simulink model "CrCtl_Governor"  (R2016b)
settings: configuration reference "CodeGenConfigSet" (kept outside this file)
values from neighbouring files (symbols this model uses):
  ACC_ZERO = fi(0,Acc_m_s2)    [init_CrCtl_Governor.m]
  CrCtl_facAcc2TrqCor_C = Calibration.Parameter    [init_CrCtl_Governor.m]
  CrCtl_facDecl2TrqCor_C = Calibration.Parameter    [init_CrCtl_Governor.m]
  CrCtl_facPT11_C = Calibration.Parameter    [init_CrCtl_Governor.m]
  CrCtl_facPT12_C = Calibration.Parameter    [init_CrCtl_Governor.m]
  CrCtl_facPT13_C = Calibration.Parameter    [init_CrCtl_Governor.m]
  CrCtl_facRmpSlpHiAcc_C = Calibration.Parameter    [init_CrCtl_Governor.m]
  CrCtl_facRmpSlpHiDecl_C = Calibration.Parameter    [init_CrCtl_Governor.m]
  CrCtl_facSlpConstRmpDwn_C = Calibration.Parameter    [init_CrCtl_Governor.m]
  CrCtl_facSlpConstRmpUp_C = Calibration.Parameter    [init_CrCtl_Governor.m]
  CrCtl_facSlpRmp1Sus_C = Calibration.Parameter    [init_CrCtl_Governor.m]
  CrCtl_facSlpRmp2Sus_C = Calibration.Parameter    [init_CrCtl_Governor.m]
  CrCtl_facTipDwnCor_CUR = Calibration.Parameter    [init_CrCtl_Governor.m]
  CrCtl_facTipDwnCor_CURX = Calibration.Parameter    [init_CrCtl_Governor.m]
  CrCtl_facTipUpCor_CUR = Calibration.Parameter    [init_CrCtl_Governor.m]
  CrCtl_facTipUpCor_CURX = Calibration.Parameter    [init_CrCtl_Governor.m]
  CrCtl_facTrqIncrSlpConstRmp_C = Calibration.Parameter    [init_CrCtl_Governor.m]
  CrCtl_facTrqIncrTimeConstRmp_C = Calibration.Parameter    [init_CrCtl_Governor.m]
  CrCtl_facTrqRedSlpConstRmp_C = Calibration.Parameter    [init_CrCtl_Governor.m]
  CrCtl_facTrqRedTimeConstRmp_C = Calibration.Parameter    [init_CrCtl_Governor.m]
  CrCtl_facTrqStrtAcc_C = Calibration.Parameter    [init_CrCtl_Governor.m]
  CrCtl_KiAcc1IWin_C = Calibration.Parameter    [init_CrCtl_Governor.m]
  CrCtl_KiAcc2IWin_C = Calibration.Parameter    [init_CrCtl_Governor.m]
  CrCtl_KiAcc3IWin_C = Calibration.Parameter    [init_CrCtl_Governor.m]
  CrCtl_KiCruise1IWin_C = Calibration.Parameter    [init_CrCtl_Governor.m]
  CrCtl_KiCruise2IWin_C = Calibration.Parameter    [init_CrCtl_Governor.m]
  CrCtl_KiCruise3IWin_C = Calibration.Parameter    [init_CrCtl_Governor.m]
  CrCtl_KiDecl1IWin_C = Calibration.Parameter    [init_CrCtl_Governor.m]
  CrCtl_KiDecl2IWin_C = Calibration.Parameter    [init_CrCtl_Governor.m]
  CrCtl_KiDecl3IWin_C = Calibration.Parameter    [init_CrCtl_Governor.m]
  CrCtl_KiNegAcc1IWin_C = Calibration.Parameter    [init_CrCtl_Governor.m]
  CrCtl_KiNegAcc2IWin_C = Calibration.Parameter    [init_CrCtl_Governor.m]
  CrCtl_KiNegAcc3IWin_C = Calibration.Parameter    [init_CrCtl_Governor.m]
  CrCtl_KiNegCruise1IWin_C = Calibration.Parameter    [init_CrCtl_Governor.m]
  CrCtl_KiNegCruise2IWin_C = Calibration.Parameter    [init_CrCtl_Governor.m]
  CrCtl_KiNegCruise3IWin_C = Calibration.Parameter    [init_CrCtl_Governor.m]
  CrCtl_KiNegDecl1IWin_C = Calibration.Parameter    [init_CrCtl_Governor.m]
  CrCtl_KiNegDecl2IWin_C = Calibration.Parameter    [init_CrCtl_Governor.m]
  CrCtl_KiNegDecl3IWin_C = Calibration.Parameter    [init_CrCtl_Governor.m]
  CrCtl_KiNegRes1IWin_C = Calibration.Parameter    [init_CrCtl_Governor.m]
  CrCtl_KiNegRes2IWin_C = Calibration.Parameter    [init_CrCtl_Governor.m]
  CrCtl_KiNegRes3IWin_C = Calibration.Parameter    [init_CrCtl_Governor.m]
  CrCtl_KiNegResCruise1IWin_C = Calibration.Parameter    [init_CrCtl_Governor.m]
  CrCtl_KiNegResCruise2IWin_C = Calibration.Parameter    [init_CrCtl_Governor.m]
  CrCtl_KiNegResCruise3IWin_C = Calibration.Parameter    [init_CrCtl_Governor.m]
  CrCtl_KiPosAcc1IWin_C = Calibration.Parameter    [init_CrCtl_Governor.m]
  CrCtl_KiPosAcc2IWin_C = Calibration.Parameter    [init_CrCtl_Governor.m]
  CrCtl_KiPosAcc3IWin_C = Calibration.Parameter    [init_CrCtl_Governor.m]
  CrCtl_KiPosCruise1IWin_C = Calibration.Parameter    [init_CrCtl_Governor.m]
  CrCtl_KiPosCruise2IWin_C = Calibration.Parameter    [init_CrCtl_Governor.m]
  CrCtl_KiPosCruise3IWin_C = Calibration.Parameter    [init_CrCtl_Governor.m]
  CrCtl_KiPosDecl1IWin_C = Calibration.Parameter    [init_CrCtl_Governor.m]
  CrCtl_KiPosDecl2IWin_C = Calibration.Parameter    [init_CrCtl_Governor.m]
  CrCtl_KiPosDecl3IWin_C = Calibration.Parameter    [init_CrCtl_Governor.m]
  CrCtl_KiPosRes1IWin_C = Calibration.Parameter    [init_CrCtl_Governor.m]
  CrCtl_KiPosRes3IWin_C = Calibration.Parameter    [init_CrCtl_Governor.m]
  CrCtl_KiPosResCruise1IWin_C = Calibration.Parameter    [init_CrCtl_Governor.m]
  CrCtl_KiPosResCruise2IWin_C = Calibration.Parameter    [init_CrCtl_Governor.m]
  CrCtl_KiPosResCruise3IWin_C = Calibration.Parameter    [init_CrCtl_Governor.m]
  CrCtl_KiRes1IWin_C = Calibration.Parameter    [init_CrCtl_Governor.m]
  CrCtl_KiRes2IWin_C = Calibration.Parameter    [init_CrCtl_Governor.m]
  CrCtl_KiRes3IWin_C = Calibration.Parameter    [init_CrCtl_Governor.m]
  CrCtl_KiResCruise1IWin_C = Calibration.Parameter    [init_CrCtl_Governor.m]
  CrCtl_KiResCruise2IWin_C = Calibration.Parameter    [init_CrCtl_Governor.m]
  CrCtl_KiResCruise3IWin_C = Calibration.Parameter    [init_CrCtl_Governor.m]
  CrCtl_KpAcc1PWin_C = Calibration.Parameter    [init_CrCtl_Governor.m]
  CrCtl_KpAcc2PWin_C = Calibration.Parameter    [init_CrCtl_Governor.m]
  CrCtl_KpAcc3PWin_C = Calibration.Parameter    [init_CrCtl_Governor.m]
  CrCtl_KpCruise1PWin_C = Calibration.Parameter    [init_CrCtl_Governor.m]
  CrCtl_KpCruise2PWin_C = Calibration.Parameter    [init_CrCtl_Governor.m]
  CrCtl_KpCruise3PWin_C = Calibration.Parameter    [init_CrCtl_Governor.m]
  CrCtl_KpDecl1PWin_C = Calibration.Parameter    [init_CrCtl_Governor.m]
  CrCtl_KpDecl2PWin_C = Calibration.Parameter    [init_CrCtl_Governor.m]
  CrCtl_KpDecl3PWin_C = Calibration.Parameter    [init_CrCtl_Governor.m]
  CrCtl_KpNegAcc1PWin_C = Calibration.Parameter    [init_CrCtl_Governor.m]
  CrCtl_KpNegAcc2PWin_C = Calibration.Parameter    [init_CrCtl_Governor.m]
  CrCtl_KpNegAcc3PWin_C = Calibration.Parameter    [init_CrCtl_Governor.m]
  CrCtl_KpNegCruise1PWin_C = Calibration.Parameter    [init_CrCtl_Governor.m]
  CrCtl_KpNegCruise2PWin_C = Calibration.Parameter    [init_CrCtl_Governor.m]
  CrCtl_KpNegCruise3PWin_C = Calibration.Parameter    [init_CrCtl_Governor.m]
  CrCtl_KpNegDecl1PWin_C = Calibration.Parameter    [init_CrCtl_Governor.m]
  CrCtl_KpNegDecl2PWin_C = Calibration.Parameter    [init_CrCtl_Governor.m]
  CrCtl_KpNegDecl3PWin_C = Calibration.Parameter    [init_CrCtl_Governor.m]
  CrCtl_KpNegRes1PWin_C = Calibration.Parameter    [init_CrCtl_Governor.m]
  CrCtl_KpNegRes2PWin_C = Calibration.Parameter    [init_CrCtl_Governor.m]
  CrCtl_KpNegRes3PWin_C = Calibration.Parameter    [init_CrCtl_Governor.m]
  CrCtl_KpNegResCruise1PWin_C = Calibration.Parameter    [init_CrCtl_Governor.m]
  CrCtl_KpNegResCruise2PWin_C = Calibration.Parameter    [init_CrCtl_Governor.m]
  CrCtl_KpNegResCruise3PWin_C = Calibration.Parameter    [init_CrCtl_Governor.m]
  CrCtl_KpPosAcc1PWin_C = Calibration.Parameter    [init_CrCtl_Governor.m]
  CrCtl_KpPosAcc2PWin_C = Calibration.Parameter    [init_CrCtl_Governor.m]
  CrCtl_KpPosAcc3PWin_C = Calibration.Parameter    [init_CrCtl_Governor.m]
  CrCtl_KpPosCruise1PWin_C = Calibration.Parameter    [init_CrCtl_Governor.m]
  CrCtl_KpPosCruise2PWin_C = Calibration.Parameter    [init_CrCtl_Governor.m]
  CrCtl_KpPosCruise3PWin_C = Calibration.Parameter    [init_CrCtl_Governor.m]
  CrCtl_KpPosDecl1PWin_C = Calibration.Parameter    [init_CrCtl_Governor.m]
  CrCtl_KpPosDecl2PWin_C = Calibration.Parameter    [init_CrCtl_Governor.m]
  CrCtl_KpPosDecl3PWin_C = Calibration.Parameter    [init_CrCtl_Governor.m]
  CrCtl_KpPosRes1PWin_C = Calibration.Parameter    [init_CrCtl_Governor.m]
  CrCtl_KpPosRes2PWin_C = Calibration.Parameter    [init_CrCtl_Governor.m]
  CrCtl_KpPosRes3PWin_C = Calibration.Parameter    [init_CrCtl_Governor.m]
  CrCtl_KpPosResCruise1PWin_C = Calibration.Parameter    [init_CrCtl_Governor.m]
  CrCtl_KpPosResCruise2PWin_C = Calibration.Parameter    [init_CrCtl_Governor.m]
  CrCtl_KpPosResCruise3PWin_C = Calibration.Parameter    [init_CrCtl_Governor.m]
  CrCtl_KpRes1PWin_C = Calibration.Parameter    [init_CrCtl_Governor.m]
  CrCtl_KpRes2PWin_C = Calibration.Parameter    [init_CrCtl_Governor.m]
  CrCtl_KpRes3PWin_C = Calibration.Parameter    [init_CrCtl_Governor.m]
  CrCtl_KpResCruise1PWin_C = Calibration.Parameter    [init_CrCtl_Governor.m]
  CrCtl_KpResCruise2PWin_C = Calibration.Parameter    [init_CrCtl_Governor.m]
  CrCtl_KpResCruise3PWin_C = Calibration.Parameter    [init_CrCtl_Governor.m]
  CrCtl_numParSelThres1_C = Calibration.Parameter    [init_CrCtl_Governor.m]
  CrCtl_numParSelThres2_C = Calibration.Parameter    [init_CrCtl_Governor.m]
  CrCtl_swtBrkMode_C = Calibration.Parameter    [init_CrCtl_Governor.m]
  CrCtl_swtILimWithP_C = Calibration.Parameter    [init_CrCtl_Governor.m]
  CrCtl_swtOvrRdeFrzInteg_C = Calibration.Parameter    [init_CrCtl_Governor.m]
  CrCtl_swtParSelHysBrk_C = Calibration.Parameter    [init_CrCtl_Governor.m]
  CrCtl_swtPT1EngBrk_C = Calibration.Parameter    [init_CrCtl_Governor.m]
  CrCtl_swtSusRmpInit_C = Calibration.Parameter    [init_CrCtl_Governor.m]
  CrCtl_swtSusRmpStp_C = Calibration.Parameter    [init_CrCtl_Governor.m]
  CrCtl_swtTipUpDwnGvnrStrtVal_C = Calibration.Parameter    [init_CrCtl_Governor.m]
  ... (+88 more)
undefined symbols (not defined in the file or in its folder): CrCtl_Governor_DT, CrCtl_stLck_conv, CrCtl_stOpFunc_conv, CrCtl_stShOff_conv, CrCtl_stSub_conv, CrCtl_stSuspRamp_conv, CruiseCtl_State_conv, EBrk_stPreSelMode_conv, WESDem_State_conv
libraries: CXLib x126, simulink x25
(part 2 of 6)

== system CrCtl_Governor/OFF State ==
  CrCtl_trqLimAct : Inport
  CrCtl_trqMin : Inport  Port=2
  CrCtl_stShOff : Inport  Port=3
  PT_trqWhlMinEng : Inport  Port=4
  CrCtl_trqReqOld : Inport  Port=5
  CrCtl_stSubGvnr : Inport  Port=6
  CrCtl_st : Inport  Port=7
  CrCtl_stSub : Inport  Port=8
  CrCtl_stLck : Inport  Port=9
  Enable : EnablePort
  CRCTL_SUBRMP : Subsystem
  "CRCTL_SUBSTRTVAL " : Subsystem
  Constant1 : Constant  Value=CrCtl_stSub_conv.CRCTL_SUBRMP
  Constant2 : Constant  Value=CrCtl_stSub_conv.CRCTL_SUBSTRTVAL
  Merge : Merge
  Relational Operator1 : RelationalOperator  Operator===  OutDataTypeStr=boolean  RndMeth=Simplest
  Relational Operator2 : RelationalOperator  Operator===  OutDataTypeStr=boolean  RndMeth=Simplest
  Terminator : Terminator
  Terminator1 : Terminator
  Terminator2 : Terminator
  CrCtl_trqReq : Outport
  wires:
  CrCtl_trqLimAct/1 -> CRCTL_SUBRMP/4(CrCtl_trqLimAct), "CRCTL_SUBSTRTVAL "/1(CrCtl_trqLimAct)
  CrCtl_trqMin/1 -> CRCTL_SUBRMP/5(CrCtl_trqMin), "CRCTL_SUBSTRTVAL "/2(CrCtl_trqMin)
  Constant2/1 -> Relational Operator2/2
  Relational Operator2/1 -> "CRCTL_SUBSTRTVAL "/Enable
  CrCtl_stSubGvnr/1 -> Relational Operator1/1, Relational Operator2/1
  Constant1/1 -> Relational Operator1/2
  Relational Operator1/1 -> CRCTL_SUBRMP/Enable
  CrCtl_st/1 -> CRCTL_SUBRMP/1(CrCtl_st)
  CrCtl_stSub/1 -> CRCTL_SUBRMP/2(CrCtl_stSub)
  CrCtl_stLck/1 -> CRCTL_SUBRMP/3(CrCtl_stLck)
  Merge/1 -> CrCtl_trqReq/1
  "CRCTL_SUBSTRTVAL "/1(CrCtl_trqReq) -> Merge/1
  CRCTL_SUBRMP/4(CrCtl_trqReq) -> Merge/2
  CRCTL_SUBRMP/1(CrCtl_st_mp) -> Terminator/1
  CRCTL_SUBRMP/3(CrCtl_stLck_mp) -> Terminator2/1
  CRCTL_SUBRMP/2(CrCtl_stSub_mp) -> Terminator1/1
  PT_trqWhlMinEng/1 -> CRCTL_SUBRMP/7(PT_trqWhlMinEng)
  CrCtl_stShOff/1 -> CRCTL_SUBRMP/6(CrCtl_stShOff)
  CrCtl_trqReqOld/1 -> "CRCTL_SUBSTRTVAL "/3(CrCtl_trqReqOld), CRCTL_SUBRMP/8(CrCtl_trqReqOld)

== system CrCtl_Governor/Operating Status Cruise Control ==
  CrCtl_stGvnr : Inport
  CrCtl_stSubGvnr : Inport  Port=2
  CrCtl_stShOff : Inport  Port=3
  CrCtl_stIWin_mp : Inport  Port=4
  Bitwise Operator : simulink/Logic and Bit Operations/Bitwise Operator  logicop=AND  UseBitMask=on  BitMask=bin2dec('00000010')  BitMaskRealWorld=Stored Integer
  Constant : Constant  Value=CrCtl_stShOff_conv.CRCTL_CUT
  Constant1 : Constant  Value=CruiseCtl_State_conv.CrCtl_STAND_BY
  Constant2 : Constant  Value=CruiseCtl_State_conv.CrCtl_ERROR
  Constant3 : Constant  Value=CrCtl_stSub_conv.CRCTL_SUBNOSUB
  Constant4 : Constant  Value=CrCtl_stOpFunc_conv.CRCTL_NOTACTV
  Constant5 : Constant  Value=CrCtl_stOpFunc_conv.CRCTL_ACTV
  Constant6 : Constant  Value=CrCtl_stOpFunc_conv.CRCTL_OVERRIDE
  Constant7 : Constant  Value=CruiseCtl_State_conv.CrCtl_STAND_BY
  Constant9 : Constant  Value=CrCtl_stSub_conv.CRCTL_SUBNOSUB
  Logical Operator : Logic  AllPortsSameDT=off  OutDataTypeStr=boolean
  Logical Operator1 : Logic  Inputs=3  AllPortsSameDT=off  OutDataTypeStr=boolean
  Logical Operator2 : Logic  AllPortsSameDT=off  OutDataTypeStr=boolean
  Logical Operator3 : Logic  Inputs=3  AllPortsSameDT=off  OutDataTypeStr=boolean
  Relational Operator{,1..3} (4 alike) : RelationalOperator  Operator=~=  OutDataTypeStr=boolean  RndMeth=Simplest
  Relational Operator4 : RelationalOperator  Operator===  OutDataTypeStr=boolean  RndMeth=Simplest
  Relational Operator5 : RelationalOperator  Operator===  OutDataTypeStr=boolean  RndMeth=Simplest
  Switch : Switch  Criteria=u2 ~= 0
  Switch1 : Switch  Criteria=u2 ~= 0
  CrCtl_stReq : Outport
  CrCtl_stPtd : Outport  Port=2
  CrCtl_stOpFunc : Outport  Port=3
  wires:
  Constant1/1 -> Relational Operator/2
  Constant2/1 -> Relational Operator1/2
  CrCtl_stSubGvnr/1 -> Relational Operator5/1, Relational Operator2/1
  Constant3/1 -> Relational Operator2/2
  CrCtl_stShOff/1 -> Relational Operator3/1
  Constant/1 -> Relational Operator3/2
  Relational Operator/1 -> Logical Operator/1
  Relational Operator1/1 -> Logical Operator3/1, Logical Operator/2
  Logical Operator/1 -> Logical Operator1/1
  Relational Operator3/1 -> Logical Operator3/3, Logical Operator1/3
  Logical Operator1/1 -> CrCtl_stReq/1
  CrCtl_stIWin_mp/1 -> Bitwise Operator/1
  Bitwise Operator/1 -> Switch/2
  Constant6/1 -> Switch/1
  Switch1/1 -> Switch/3
  Switch/1 -> CrCtl_stOpFunc/1
  CrCtl_stGvnr/1 -> Relational Operator4/1, Relational Operator1/1, Relational Operator/1
  Constant7/1 -> Relational Operator4/2
  Relational Operator4/1 -> Logical Operator2/1
  Relational Operator5/1 -> Logical Operator2/2
  Constant9/1 -> Relational Operator5/2
  Logical Operator2/1 -> Switch1/2
  Constant4/1 -> Switch1/1
  Constant5/1 -> Switch1/3
  Relational Operator2/1 -> Logical Operator3/2, Logical Operator1/2
  Logical Operator3/1 -> CrCtl_stPtd/1

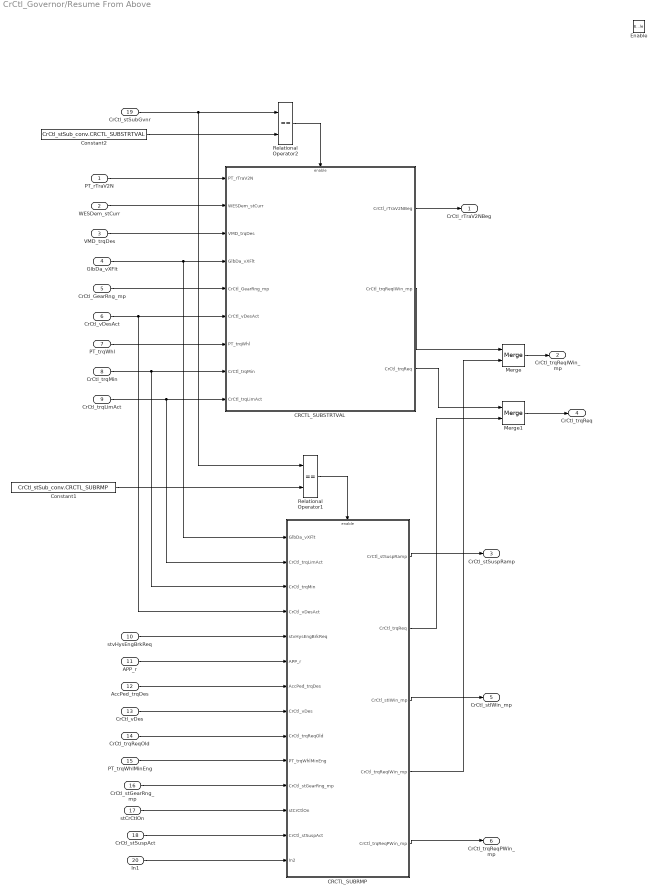
== system CrCtl_Governor/Resume From Above ==
  PT_rTraV2N : Inport
  WESDem_stCurr : Inport  Port=2
  VMD_trqDes : Inport  Port=3
  GlbDa_vXFlt : Inport  Port=4
  CrCtl_GearRng_mp : Inport  Port=5
  CrCtl_vDesAct : Inport  Port=6
  PT_trqWhl : Inport  Port=7
  CrCtl_trqMin : Inport  Port=8
  CrCtl_trqLimAct : Inport  Port=9
  stvHysEngBrkReq : Inport  Port=10
  APP_r : Inport  Port=11
  AccPed_trqDes : Inport  Port=12
  CrCtl_vDes : Inport  Port=13
  CrCtl_trqReqOld : Inport  Port=14
  PT_trqWhlMinEng : Inport  Port=15
  CrCtl_stGearRng_mp : Inport  Port=16
  stCrCtlOn : Inport  Port=17
  CrCtl_stSuspAct : Inport  Port=18
  CrCtl_stSubGvnr : Inport  Port=19
  In1 : Inport  Port=20
  Enable : EnablePort
  CRCTL_SUBRMP : Subsystem
  CRCTL_SUBSTRTVAL : Subsystem
  Constant1 : Constant  Value=CrCtl_stSub_conv.CRCTL_SUBRMP
  Constant2 : Constant  Value=CrCtl_stSub_conv.CRCTL_SUBSTRTVAL
  Merge : Merge
  Merge1 : Merge
  Relational Operator1 : RelationalOperator  Operator===  OutDataTypeStr=boolean  RndMeth=Simplest
  Relational Operator2 : RelationalOperator  Operator===  OutDataTypeStr=boolean  RndMeth=Simplest
  CrCtl_rTraV2NBeg : Outport
  CrCtl_trqReqIWin_mp : Outport  Port=2
  CrCtl_stSuspRamp : Outport  Port=3
  CrCtl_trqReq : Outport  Port=4
  CrCtl_stIWin_mp : Outport  Port=5
  CrCtl_trqReqPWin_mp : Outport  Port=6
  wires:
  PT_rTraV2N/1 -> CRCTL_SUBSTRTVAL/1(PT_rTraV2N)
  WESDem_stCurr/1 -> CRCTL_SUBSTRTVAL/2(WESDem_stCurr)
  VMD_trqDes/1 -> CRCTL_SUBSTRTVAL/3(VMD_trqDes)
  GlbDa_vXFlt/1 -> CRCTL_SUBRMP/1(GlbDa_vXFlt), CRCTL_SUBSTRTVAL/4(GlbDa_vXFlt)
  CrCtl_GearRng_mp/1 -> CRCTL_SUBSTRTVAL/5(CrCtl_GearRng_mp)
  CrCtl_trqLimAct/1 -> CRCTL_SUBRMP/2(CrCtl_trqLimAct), CRCTL_SUBSTRTVAL/9(CrCtl_trqLimAct)
  CrCtl_trqMin/1 -> CRCTL_SUBRMP/3(CrCtl_trqMin), CRCTL_SUBSTRTVAL/8(CrCtl_trqMin)
  PT_trqWhl/1 -> CRCTL_SUBSTRTVAL/7(PT_trqWhl)
  Constant2/1 -> Relational Operator2/2
  Relational Operator2/1 -> CRCTL_SUBSTRTVAL/Enable
  CrCtl_stSubGvnr/1 -> Relational Operator1/1, Relational Operator2/1
  Constant1/1 -> Relational Operator1/2
  Relational Operator1/1 -> CRCTL_SUBRMP/Enable
  CrCtl_vDesAct/1 -> CRCTL_SUBRMP/4(CrCtl_vDesAct), CRCTL_SUBSTRTVAL/6(CrCtl_vDesAct)
  stvHysEngBrkReq/1 -> CRCTL_SUBRMP/5(stvHysEngBrkReq)
  APP_r/1 -> CRCTL_SUBRMP/6(APP_r)
  AccPed_trqDes/1 -> CRCTL_SUBRMP/7(AccPed_trqDes)
  stCrCtlOn/1 -> CRCTL_SUBRMP/12(stCrCtlOn)
  CrCtl_stGearRng_mp/1 -> CRCTL_SUBRMP/11(CrCtl_stGearRng_mp)
  PT_trqWhlMinEng/1 -> CRCTL_SUBRMP/10(PT_trqWhlMinEng)
  CrCtl_vDes/1 -> CRCTL_SUBRMP/8(CrCtl_vDes)
  CrCtl_stSuspAct/1 -> CRCTL_SUBRMP/13(CrCtl_stSuspAct)
  CrCtl_trqReqOld/1 -> CRCTL_SUBRMP/9(CrCtl_trqReqOld)
  CRCTL_SUBSTRTVAL/1(CrCtl_rTraV2NBeg) -> CrCtl_rTraV2NBeg/1
  CRCTL_SUBRMP/2(CrCtl_trqReq) -> Merge1/2
  CRCTL_SUBRMP/3(CrCtl_stIWin_mp) -> CrCtl_stIWin_mp/1
  CRCTL_SUBRMP/1(CrCtl_stSuspRamp) -> CrCtl_stSuspRamp/1
  CRCTL_SUBRMP/4(CrCtl_trqReqIWin_mp) -> Merge/2
  Merge/1 -> CrCtl_trqReqIWin_mp/1
  CRCTL_SUBSTRTVAL/2(CrCtl_trqReqIWin_mp) -> Merge/1
  CRCTL_SUBSTRTVAL/3(CrCtl_trqReq) -> Merge1/1
  Merge1/1 -> CrCtl_trqReq/1
  CRCTL_SUBRMP/5(CrCtl_trqReqPWin_mp) -> CrCtl_trqReqPWin_mp/1
  In1/1 -> CRCTL_SUBRMP/14(In2)

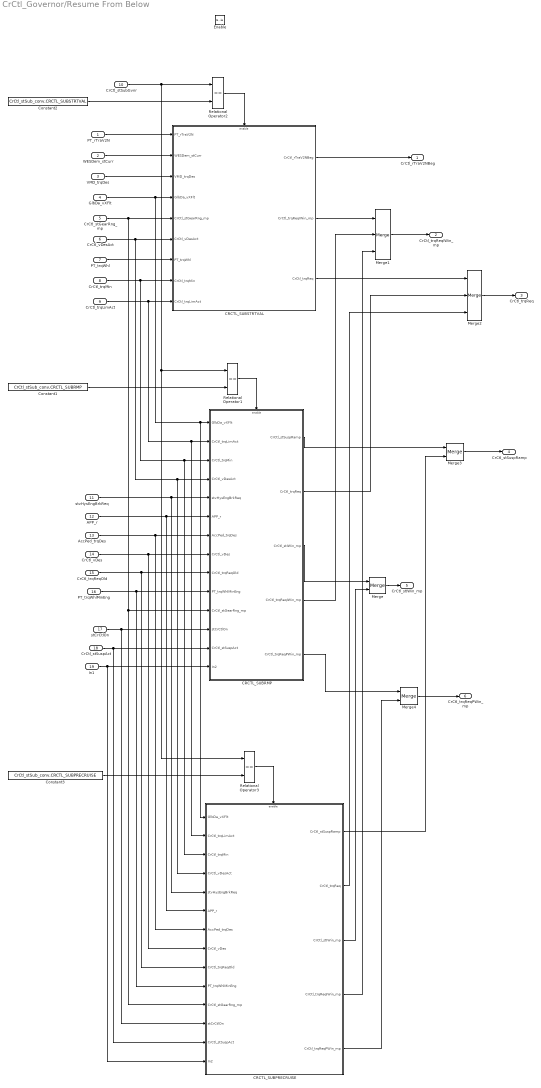
== system CrCtl_Governor/Resume From Below ==
  PT_rTraV2N : Inport
  WESDem_stCurr : Inport  Port=2
  VMD_trqDes : Inport  Port=3
  GlbDa_vXFlt : Inport  Port=4
  CrCtl_stGearRng_mp : Inport  Port=5
  CrCtl_vDesAct : Inport  Port=6
  PT_trqWhl : Inport  Port=7
  CrCtl_trqMin : Inport  Port=8
  CrCtl_trqLimAct : Inport  Port=9
  CrCtl_stSubGvnr : Inport  Port=10
  stvHysEngBrkReq : Inport  Port=11
  APP_r : Inport  Port=12
  AccPed_trqDes : Inport  Port=13
  CrCtl_vDes : Inport  Port=14
  CrCtl_trqReqOld : Inport  Port=15
  PT_trqWhlMinEng : Inport  Port=16
  stCrCtlOn : Inport  Port=17
  CrCtl_stSuspAct : Inport  Port=18
  In1 : Inport  Port=19
  Enable : EnablePort
  CRCTL_SUBPRECRUISE : Subsystem
  CRCTL_SUBRMP : Subsystem
  CRCTL_SUBSTRTVAL : Subsystem
  Constant1 : Constant  Value=CrCtl_stSub_conv.CRCTL_SUBRMP
  Constant2 : Constant  Value=CrCtl_stSub_conv.CRCTL_SUBSTRTVAL
  Constant3 : Constant  Value=CrCtl_stSub_conv.CRCTL_SUBPRECRUISE
  Merge : Merge
  Merge1 : Merge  Inputs=3
  Merge2 : Merge  Inputs=3
  Merge3 : Merge
  Merge4 : Merge
  Relational Operator1 : RelationalOperator  Operator===  OutDataTypeStr=boolean  RndMeth=Simplest
  Relational Operator2 : RelationalOperator  Operator===  OutDataTypeStr=boolean  RndMeth=Simplest
  Relational Operator3 : RelationalOperator  Operator===  OutDataTypeStr=boolean  RndMeth=Simplest
  CrCtl_rTraV2NBeg : Outport
  CrCtl_trqReqIWin_mp : Outport  Port=2
  CrCtl_trqReq : Outport  Port=3
  CrCtl_stSuspRamp : Outport  Port=4
  CrCtl_stIWin_mp : Outport  Port=5
  CrCtl_trqReqPWin_mp : Outport  Port=6
  wires:
  PT_rTraV2N/1 -> CRCTL_SUBSTRTVAL/1(PT_rTraV2N)
  WESDem_stCurr/1 -> CRCTL_SUBSTRTVAL/2(WESDem_stCurr)
  VMD_trqDes/1 -> CRCTL_SUBSTRTVAL/3(VMD_trqDes)
  GlbDa_vXFlt/1 -> CRCTL_SUBPRECRUISE/1(GlbDa_vXFlt), CRCTL_SUBRMP/1(GlbDa_vXFlt), CRCTL_SUBSTRTVAL/4(GlbDa_vXFlt)
  CrCtl_trqLimAct/1 -> CRCTL_SUBPRECRUISE/2(CrCtl_trqLimAct), CRCTL_SUBRMP/2(CrCtl_trqLimAct), CRCTL_SUBSTRTVAL/9(CrCtl_trqLimAct)
  CrCtl_trqMin/1 -> CRCTL_SUBPRECRUISE/3(CrCtl_trqMin), CRCTL_SUBRMP/3(CrCtl_trqMin), CRCTL_SUBSTRTVAL/8(CrCtl_trqMin)
  PT_trqWhl/1 -> CRCTL_SUBSTRTVAL/7(PT_trqWhl)
  Constant2/1 -> Relational Operator2/2
  Relational Operator2/1 -> CRCTL_SUBSTRTVAL/Enable
  Constant1/1 -> Relational Operator1/2
  Relational Operator1/1 -> CRCTL_SUBRMP/Enable
  CrCtl_stSubGvnr/1 -> Relational Operator3/1, Relational Operator1/1, Relational Operator2/1
  Constant3/1 -> Relational Operator3/2
  Relational Operator3/1 -> CRCTL_SUBPRECRUISE/Enable
  CrCtl_vDesAct/1 -> CRCTL_SUBPRECRUISE/4(CrCtl_vDesAct), CRCTL_SUBRMP/4(CrCtl_vDesAct), CRCTL_SUBSTRTVAL/6(CrCtl_vDesAct)
  stvHysEngBrkReq/1 -> CRCTL_SUBPRECRUISE/5(stvHysEngBrkReq), CRCTL_SUBRMP/5(stvHysEngBrkReq)
  APP_r/1 -> CRCTL_SUBPRECRUISE/6(APP_r), CRCTL_SUBRMP/6(APP_r)
  AccPed_trqDes/1 -> CRCTL_SUBPRECRUISE/7(AccPed_trqDes), CRCTL_SUBRMP/7(AccPed_trqDes)
  stCrCtlOn/1 -> CRCTL_SUBPRECRUISE/12(stCrCtlOn), CRCTL_SUBRMP/12(stCrCtlOn)
  CrCtl_stGearRng_mp/1 -> CRCTL_SUBPRECRUISE/11(CrCtl_stGearRng_mp), CRCTL_SUBRMP/11(CrCtl_stGearRng_mp), CRCTL_SUBSTRTVAL/5(CrCtl_stGearRng_mp)
  PT_trqWhlMinEng/1 -> CRCTL_SUBPRECRUISE/10(PT_trqWhlMinEng), CRCTL_SUBRMP/10(PT_trqWhlMinEng)
  CrCtl_vDes/1 -> CRCTL_SUBPRECRUISE/8(CrCtl_vDes), CRCTL_SUBRMP/8(CrCtl_vDes)
  CrCtl_stSuspAct/1 -> CRCTL_SUBPRECRUISE/13(CrCtl_stSuspAct), CRCTL_SUBRMP/13(CrCtl_stSuspAct)
  CrCtl_trqReqOld/1 -> CRCTL_SUBPRECRUISE/9(CrCtl_trqReqOld), CRCTL_SUBRMP/9(CrCtl_trqReqOld)
  Merge3/1 -> CrCtl_stSuspRamp/1
  Merge/1 -> CrCtl_stIWin_mp/1
  CRCTL_SUBSTRTVAL/1(CrCtl_rTraV2NBeg) -> CrCtl_rTraV2NBeg/1
  Merge2/1 -> CrCtl_trqReq/1
  CRCTL_SUBSTRTVAL/3(CrCtl_trqReq) -> Merge2/1
  Merge1/1 -> CrCtl_trqReqIWin_mp/1
  CRCTL_SUBSTRTVAL/2(CrCtl_trqReqIWin_mp) -> Merge1/1
  CRCTL_SUBRMP/3(CrCtl_stIWin_mp) -> Merge/1
  CRCTL_SUBPRECRUISE/3(CrCtl_stIWin_mp) -> Merge/2
  CRCTL_SUBRMP/1(CrCtl_stSuspRamp) -> Merge3/1
  CRCTL_SUBPRECRUISE/1(CrCtl_stSuspRamp) -> Merge3/2
  CRCTL_SUBRMP/2(CrCtl_trqReq) -> Merge2/2
  CRCTL_SUBRMP/4(CrCtl_trqReqIWin_mp) -> Merge1/2
  CRCTL_SUBPRECRUISE/2(CrCtl_trqReq) -> Merge2/3
  CRCTL_SUBPRECRUISE/4(CrCtl_trqReqIWin_mp) -> Merge1/3
  Merge4/1 -> CrCtl_trqReqPWin_mp/1
  CRCTL_SUBRMP/5(CrCtl_trqReqPWin_mp) -> Merge4/1
  CRCTL_SUBPRECRUISE/5(CrCtl_trqReqPWin_mp) -> Merge4/2
  In1/1 -> CRCTL_SUBPRECRUISE/14(In2), CRCTL_SUBRMP/14(In2)

== system CrCtl_Governor/STAND BY State ==
  PT_trqWhlMinEng : Inport
  Enable : EnablePort
  CrCtl_trqReq : Outport
  wires:
  PT_trqWhlMinEng/1 -> CrCtl_trqReq/1

== system CrCtl_Governor/Subsystem ==
  Constant : Constant  Value=0  OutDataTypeStr=Trq_Nm
  Signal Conversion : SignalConversion  OverrideOpt=off
  Out1 : Outport
  wires:
  Constant/1 -> Signal Conversion/1
  Signal Conversion/1 -> Out1/1

== system CrCtl_Governor/Suspend Request Detection ==
  CrCtl_trqReq : Inport
  CrCtl_stSuspAct : Inport  Port=2
  Constant1 : Constant  Value=CrCtl_stSuspRamp_conv.CRCTL_SUSPENDSTARTRAMP
  Constant2 : Constant  Value=CrCtl_stSuspRamp_conv.CRCTL_SUSPENDENDRAMP
  EdgeFalling : CXLib/EdgeFalling
  EdgeRising : CXLib/EdgeRising
  Switch : Switch  Criteria=u2 ~= 0
  Switch1 : Switch  Criteria=u2 ~= 0
  Switch2 : Switch  Criteria=u2 ~= 0
  Unit Delay : UnitDelay  InitialCondition=CrCtl_stSuspRamp_conv.CRCTL_SUSPENDNOTACTIVE  SampleTime=-1
  Unit Delay1 : UnitDelay  SampleTime=-1
  CrCtl_trqReqOld : Outport
  wires:
  CrCtl_stSuspAct/1 -> Switch2/2, EdgeFalling/1, EdgeRising/1
  EdgeRising/1 -> Switch/2
  Constant1/1 -> Switch/1
  EdgeFalling/1 -> Switch1/2
  Constant2/1 -> Switch1/1
  Switch/1 -> Switch1/3
  Switch1/1 -> Unit Delay/1
  Unit Delay/1 -> Switch/3
  CrCtl_trqReq/1 -> Switch2/3
  Switch2/1 -> Unit Delay1/1, CrCtl_trqReqOld/1
  Unit Delay1/1 -> Switch2/1

== system CrCtl_Governor/Tip Down State ==
  PT_rTraV2N : Inport
  WESDem_stCurr : Inport  Port=2
  CrCtl_stSubGvnr : Inport  Port=3
  PT_trqWhlMinEng : Inport  Port=4
  CrCtl_stVDirChng : Inport  Port=5
  VMD_trqDes : Inport  Port=6
  CrCtl_vDesActOld : Inport  Port=7
  GlbDa_vXFlt : Inport  Port=8
  GlbDa_aXFlt : Inport  Port=9
  CrCtl_stGearRng_mp : Inport  Port=10
  CrCtl_vDesAct : Inport  Port=11
  PT_trqWhl : Inport  Port=12
  CrCtl_trqMin : Inport  Port=13
  CrCtl_trqLimAct : Inport  Port=14
  Enable : EnablePort
  "CRCTL_SUBCALCSET " : Subsystem
  CrCtl_rTraV2NBeg : Outport
  CrCtl_trqReq : Outport  Port=2
  CrCtl_trqReqIWin_mp : Outport  Port=3
  CrCtl_trqReqPWin_mp : Outport  Port=4
  wires:
  PT_rTraV2N/1 -> "CRCTL_SUBCALCSET "/1(PT_rTraV2N)
  WESDem_stCurr/1 -> "CRCTL_SUBCALCSET "/2(WESDem_stCurr)
  CrCtl_stSubGvnr/1 -> "CRCTL_SUBCALCSET "/3(CrCtl_stSubGvnr)
  PT_trqWhlMinEng/1 -> "CRCTL_SUBCALCSET "/4(PT_trqWhlMinEng)
  CrCtl_stVDirChng/1 -> "CRCTL_SUBCALCSET "/5(CrCtl_stVDirChng)
  VMD_trqDes/1 -> "CRCTL_SUBCALCSET "/6(VMD_trqDes)
  CrCtl_vDesActOld/1 -> "CRCTL_SUBCALCSET "/7(CrCtl_vDesActOld)
  GlbDa_vXFlt/1 -> "CRCTL_SUBCALCSET "/8(GlbDa_vXFlt)
  GlbDa_aXFlt/1 -> "CRCTL_SUBCALCSET "/9(GlbDa_aXFlt)
  CrCtl_stGearRng_mp/1 -> "CRCTL_SUBCALCSET "/10(CrCtl_stGearRng_mp)
  CrCtl_vDesAct/1 -> "CRCTL_SUBCALCSET "/11(CrCtl_vDesAct)
  PT_trqWhl/1 -> "CRCTL_SUBCALCSET "/12(PT_trqWhl)
  CrCtl_trqMin/1 -> "CRCTL_SUBCALCSET "/13(CrCtl_trqMin)
  CrCtl_trqLimAct/1 -> "CRCTL_SUBCALCSET "/14(CrCtl_trqLimAct)
  "CRCTL_SUBCALCSET "/1(CrCtl_rTraV2NBeg) -> CrCtl_rTraV2NBeg/1
  "CRCTL_SUBCALCSET "/2(CrCtl_trqReq) -> CrCtl_trqReq/1
  "CRCTL_SUBCALCSET "/3(CrCtl_trqReqIWin_mp) -> CrCtl_trqReqIWin_mp/1
  "CRCTL_SUBCALCSET "/4(CrCtl_trqReqPWin_mp) -> CrCtl_trqReqPWin_mp/1

== system CrCtl_Governor/Tip Up State ==
  PT_rTraV2N : Inport
  WESDem_stCurr : Inport  Port=2
  CrCtl_stSubGvnr : Inport  Port=3
  PT_trqWhlMinEng : Inport  Port=4
  CrCtl_stVDirChng : Inport  Port=5
  VMD_trqDes : Inport  Port=6
  CrCtl_vDesActOld : Inport  Port=7
  GlbDa_vXFlt : Inport  Port=8
  GlbDa_aXFlt : Inport  Port=9
  CrCtl_stGearRng_mp : Inport  Port=10
  CrCtl_vDesAct : Inport  Port=11
  PT_trqWhl : Inport  Port=12
  CrCtl_trqMin : Inport  Port=13
  CrCtl_trqLimAct : Inport  Port=14
  Enable : EnablePort
  Subsystem : Subsystem
  CrCtl_rTraV2NBeg : Outport
  CrCtl_trqReq : Outport  Port=2
  CrCtl_trqReqIWin_mp : Outport  Port=3
  CrCtl_trqReqPWin_mp : Outport  Port=4
  wires:
  PT_rTraV2N/1 -> Subsystem/1(PT_rTraV2N)
  WESDem_stCurr/1 -> Subsystem/2(WESDem_stCurr)
  CrCtl_stSubGvnr/1 -> Subsystem/3(CrCtl_stSubGvnr)
  PT_trqWhlMinEng/1 -> Subsystem/4(PT_trqWhlMinEng)
  CrCtl_stVDirChng/1 -> Subsystem/5(CrCtl_stVDirChng)
  VMD_trqDes/1 -> Subsystem/6(VMD_trqDes)
  CrCtl_vDesActOld/1 -> Subsystem/7(CrCtl_vDesActOld)
  GlbDa_vXFlt/1 -> Subsystem/8(GlbDa_vXFlt)
  GlbDa_aXFlt/1 -> Subsystem/9(GlbDa_aXFlt)
  CrCtl_stGearRng_mp/1 -> Subsystem/14(CrCtl_stGearRng_mp)
  CrCtl_vDesAct/1 -> Subsystem/10(CrCtl_vDesAct)
  PT_trqWhl/1 -> Subsystem/11(PT_trqWhl)
  CrCtl_trqMin/1 -> Subsystem/12(CrCtl_trqMin)
  CrCtl_trqLimAct/1 -> Subsystem/13(CrCtl_trqLimAct)
  Subsystem/1(CrCtl_rTraV2NBeg) -> CrCtl_rTraV2NBeg/1
  Subsystem/2(CrCtl_trqReq) -> CrCtl_trqReq/1
  Subsystem/3(CrCtl_trqReqIWin_mp) -> CrCtl_trqReqIWin_mp/1
  Subsystem/4(CrCtl_trqReqPWin_mp) -> CrCtl_trqReqPWin_mp/1

== system CrCtl_Governor/Working Range of Cruise Control ==
  PT_trqWhlMinEngBrk : Inport
  PT_trqWhlMinEng : Inport  Port=2
  stvHysEngBrkReq : Inport  Port=3
  EBrk_stPreSelMode : Inport  Port=4
  InjSys_trqLim : Inport  Port=5
  EngDem_trqInrLim : Inport  Port=6
  CoETS_trqUnFltLtd : Inport  Port=7
  CoETS_trqNTCActvOff : Inport  Port=8
  CoETS_trqNTCActvOn : Inport  Port=9
  RngMod_trqMin : Inport  Port=10
  PT_trqLos : Inport  Port=11
  PT_rTrq : Inport  Port=12
  VehMot_rTrqDfftl : Inport  Port=13
  CoVeh_trqAcs : Inport  Port=14
  CoVeh_trqPrpLimErr : Inport  Port=15
  Lower limiting Cruise Control torque : Subsystem
  Upper limiting Cruise Control torque : Subsystem
  CrCtl_trqMin : Outport
  CrCtl_trqLimAct : Outport  Port=2
  wires:
  Lower limiting Cruise Control torque/1(CrCtl_trqMin) -> Upper limiting Cruise Control torque/1(CrCtl_trqMin), CrCtl_trqMin/1
  PT_trqWhlMinEngBrk/1 -> Lower limiting Cruise Control torque/1(PT_trqWhlMinEngBrk)
  PT_trqWhlMinEng/1 -> Upper limiting Cruise Control torque/3(PT_trqWhlMinEng), Lower limiting Cruise Control torque/2(PT_trqWhlMinEng)
  stvHysEngBrkReq/1 -> Upper limiting Cruise Control torque/2(stvHysEngBrkReq), Lower limiting Cruise Control torque/3(stvHysEngBrkReq)
  EBrk_stPreSelMode/1 -> Lower limiting Cruise Control torque/4(EBrk_stPreSelMode)
  CoVeh_trqPrpLimErr/1 -> Upper limiting Cruise Control torque/14(CoVeh_trqPrpLimErr)
  CoVeh_trqAcs/1 -> Upper limiting Cruise Control torque/13(CoVeh_trqAcs)
  VehMot_rTrqDfftl/1 -> Upper limiting Cruise Control torque/12(VehMot_rTrqDfftl)
  PT_rTrq/1 -> Upper limiting Cruise Control torque/11(PT_rTrq)
  PT_trqLos/1 -> Upper limiting Cruise Control torque/10(PT_trqLos)
  RngMod_trqMin/1 -> Upper limiting Cruise Control torque/9(RngMod_trqMin)
  CoETS_trqNTCActvOn/1 -> Upper limiting Cruise Control torque/8(CoETS_trqNTCActvOn)
  CoETS_trqNTCActvOff/1 -> Upper limiting Cruise Control torque/7(CoETS_trqNTCActvOff)
  CoETS_trqUnFltLtd/1 -> Upper limiting Cruise Control torque/6(CoETS_trqUnFltLtd)
  EngDem_trqInrLim/1 -> Upper limiting Cruise Control torque/5(EngDem_trqInrLim)
  InjSys_trqLim/1 -> Upper limiting Cruise Control torque/4(InjSys_trqLim)
  Upper limiting Cruise Control torque/1(CrCtl_trqLimAct) -> CrCtl_trqLimAct/1

== system CrCtl_Governor/speed limiter status checking ==
  VMSLmtSwt_st : Inport
  VMSAdjBtn_st : Inport  Port=2
  CoVMD_trqLLim : Inport  Port=3
  CrCtl_trqReq : Inport  Port=4
  CrCtl_trqReqPWin_mp : Inport  Port=5
  Add : Sum  Inputs=+-
  EdgeFalling : CXLib/EdgeFalling
  EdgeFalling1 : CXLib/EdgeFalling
  Logical Operator2 : Logic  Operator=OR  AllPortsSameDT=off  OutDataTypeStr=boolean
  MinMax : MinMax  Inputs=2
  Switch : Switch  Criteria=u2 ~= 0
  Out1 : Outport
  Out2 : Outport  Port=2
  wires:
  VMSAdjBtn_st/1 -> EdgeFalling1/1
  VMSLmtSwt_st/1 -> EdgeFalling/1
  EdgeFalling/1 -> Logical Operator2/1
  EdgeFalling1/1 -> Logical Operator2/2
  CoVMD_trqLLim/1 -> MinMax/2
  Logical Operator2/1 -> Switch/2
  MinMax/1 -> Switch/1
  CrCtl_trqReq/1 -> Switch/3, MinMax/1
  CrCtl_trqReqPWin_mp/1 -> Add/2
  Switch/1 -> Add/1, Out1/1
  Add/1 -> Out2/1

== system CrCtl_Governor/Acceleration State/CRCTL_SUBPRECRUISE ==
  CrCtl_trqLimAct : Inport
  GlbDa_vXFlt : Inport  Port=2
  CrCtl_vDes : Inport  Port=3
  CrCtl_trqMin : Inport  Port=4
  CrCtl_vMaxDvtAcc : Inport  Port=5
  CrCtl_trqReqOld : Inport  Port=6
  In1 : Inport  Port=7
  Enable : EnablePort
  Add : Sum
  Constant : Constant  Value=2  OutDataTypeStr=State_uint8
  Constant1 : Constant  Value=CrCtl_facRmpSlpHiAcc_C
  Constant2 : Constant  Value=CrCtl_swtTrqLimPreCruise_C
  Constant4 : Constant  Value=CrCtl_Governor_DT
  Logical Operator : Logic  Operator=OR  AllPortsSameDT=off  OutDataTypeStr=boolean
  Logical Operator1 : Logic  Operator=OR  AllPortsSameDT=off  OutDataTypeStr=boolean
  MinMax : MinMax  Inputs=2
  Product : Product
  RAMP_S16 : CXLib/RAMP_S16
  Relational Operator : RelationalOperator  Operator=>  OutDataTypeStr=boolean  RndMeth=Simplest
  Relational Operator1 : RelationalOperator  OutDataTypeStr=boolean  RndMeth=Simplest
  Relational Operator2 : RelationalOperator  Operator===  OutDataTypeStr=boolean  RndMeth=Simplest
  Switch : Switch  Criteria=u2 ~= 0
  Switch1 : Switch  Criteria=u2 ~= 0
  Switch2 : Switch  Criteria=u2 ~= 0
  Unit Delay : UnitDelay  SampleTime=-1
  s2dt : CXLib/s2dt
  CrCtl_trqReq : Outport
  wires:
  s2dt/1 -> RAMP_S16/3, RAMP_S16/2
  Switch/1 -> s2dt/1
  Constant4/1 -> s2dt/2
  Relational Operator1/1 -> Logical Operator/1
  CrCtl_trqMin/1 -> Relational Operator2/2, RAMP_S16/1
  CrCtl_trqReqOld/1 -> RAMP_S16/5
  CrCtl_vDes/1 -> Add/1
  CrCtl_vMaxDvtAcc/1 -> Add/2
  Add/1 -> Relational Operator/2
  GlbDa_vXFlt/1 -> Relational Operator/1
  Constant/1 -> Product/2
  Relational Operator/1 -> Switch/2
  Product/1 -> Switch/1
  Constant1/1 -> Switch/3, Product/1
  CrCtl_trqLimAct/1 -> Relational Operator1/2, MinMax/1
  MinMax/1 -> Switch1/3
  Constant2/1 -> Switch2/2, Switch1/2
  RAMP_S16/1 -> Relational Operator2/1, Relational Operator1/1, Switch1/1, MinMax/2
  Relational Operator2/1 -> Switch2/1, Logical Operator/2
  Logical Operator/1 -> Switch2/3
  Switch2/1 -> Unit Delay/1
  Logical Operator1/1 -> RAMP_S16/4
  Switch1/1 -> CrCtl_trqReq/1
  In1/1 -> Logical Operator1/1
  Unit Delay/1 -> Logical Operator1/2

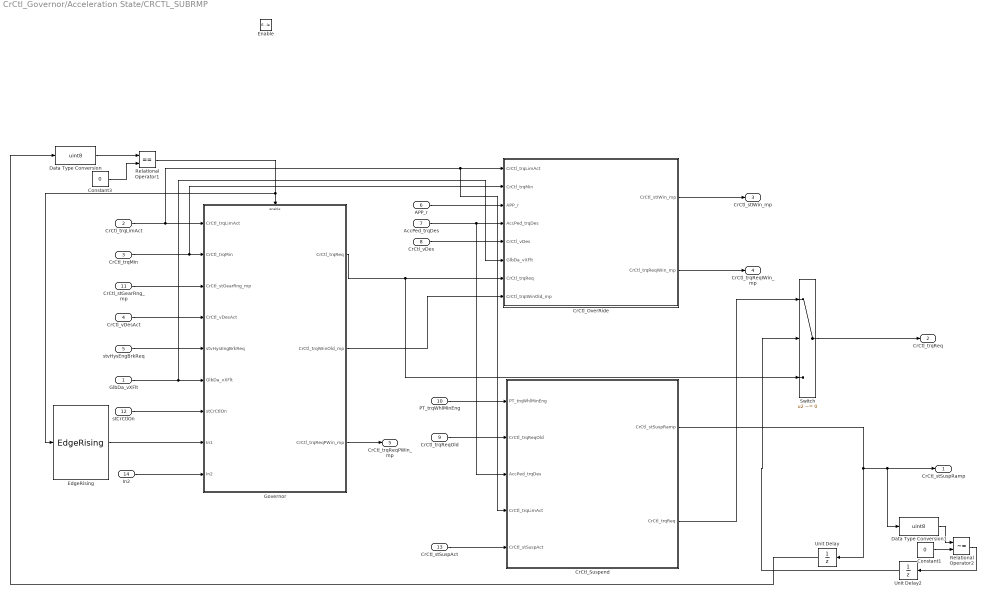
== system CrCtl_Governor/Acceleration State/CRCTL_SUBRMP ==
  GlbDa_vXFlt : Inport
  CrCtl_trqLimAct : Inport  Port=2
  CrCtl_trqMin : Inport  Port=3
  CrCtl_vDesAct : Inport  Port=4
  stvHysEngBrkReq : Inport  Port=5
  APP_r : Inport  Port=6
  AccPed_trqDes : Inport  Port=7
  CrCtl_vDes : Inport  Port=8
  CrCtl_trqReqOld : Inport  Port=9
  PT_trqWhlMinEng : Inport  Port=10
  CrCtl_stGearRng_mp : Inport  Port=11
  stCrCtlOn : Inport  Port=12
  CrCtl_stSuspAct : Inport  Port=13
  In2 : Inport  Port=14
  Enable : EnablePort
  Constant1 : Constant  Value=0  OutDataTypeStr=uint8
  Constant3 : Constant  Value=0  OutDataTypeStr=uint8
  CrCtl_OverRide : Subsystem
  CrCtl_Suspend : Subsystem
  Data Type Conversion : DataTypeConversion  OutDataTypeStr=uint8
  Data Type Conversion1 : DataTypeConversion  OutDataTypeStr=uint8
  EdgeRising : CXLib/EdgeRising
  Governor : Subsystem
  Relational Operator1 : RelationalOperator  Operator===  OutDataTypeStr=boolean  RndMeth=Simplest
  Relational Operator2 : RelationalOperator  Operator=~=  OutDataTypeStr=boolean  RndMeth=Simplest
  Switch : Switch  Criteria=u2 ~= 0
  Unit Delay : UnitDelay  InitialCondition=CrCtl_stSuspRamp_conv.CRCTL_SUSPENDNOTACTIVE  SampleTime=-1
  Unit Delay2 : UnitDelay  SampleTime=-1
  CrCtl_stSuspRamp : Outport
  CrCtl_trqReq : Outport  Port=2
  CrCtl_stIWin_mp : Outport  Port=3
  CrCtl_trqReqIWin_mp : Outport  Port=4
  CrCtl_trqReqPWin_mp : Outport  Port=5
  wires:
  Constant3/1 -> Relational Operator1/2
  stCrCtlOn/1 -> Governor/7(stCrCtlOn)
  stvHysEngBrkReq/1 -> Governor/5(stvHysEngBrkReq)
  CrCtl_vDesAct/1 -> Governor/4(CrCtl_vDesAct)
  CrCtl_stGearRng_mp/1 -> Governor/3(CrCtl_stGearRng_mp)
  CrCtl_trqMin/1 -> Governor/2(CrCtl_trqMin), CrCtl_OverRide/2(CrCtl_trqMin)
  APP_r/1 -> CrCtl_OverRide/3(APP_r)
  CrCtl_vDes/1 -> CrCtl_OverRide/5(CrCtl_vDes)
  GlbDa_vXFlt/1 -> Governor/6(GlbDa_vXFlt), CrCtl_OverRide/6(GlbDa_vXFlt)
  Governor/1(CrCtl_trqReq) -> Switch/3, CrCtl_OverRide/7(CrCtl_trqReq)
  Governor/2(CrCtl_trqIWinOld_mp) -> CrCtl_OverRide/8(CrCtl_trqIWinOld_mp)
  CrCtl_trqLimAct/1 -> Governor/1(CrCtl_trqLimAct), CrCtl_Suspend/4(CrCtl_trqLimAct), CrCtl_OverRide/1(CrCtl_trqLimAct)
  AccPed_trqDes/1 -> CrCtl_Suspend/3(AccPed_trqDes), CrCtl_OverRide/4(AccPed_trqDes)
  PT_trqWhlMinEng/1 -> CrCtl_Suspend/1(PT_trqWhlMinEng)
  CrCtl_trqReqOld/1 -> CrCtl_Suspend/2(CrCtl_trqReqOld)
  CrCtl_stSuspAct/1 -> CrCtl_Suspend/5(CrCtl_stSuspAct)
  CrCtl_Suspend/2(" CrCtl_trqReq") -> Switch/1
  CrCtl_Suspend/1(CrCtl_stSuspRamp) -> Unit Delay/1, Data Type Conversion1/1, CrCtl_stSuspRamp/1
  Switch/1 -> CrCtl_trqReq/1
  Constant1/1 -> Relational Operator2/2
  Relational Operator2/1 -> Unit Delay2/1
  CrCtl_OverRide/1(CrCtl_stIWin_mp) -> CrCtl_stIWin_mp/1
  CrCtl_OverRide/2(CrCtl_trqReqIWin_mp) -> CrCtl_trqReqIWin_mp/1
  Data Type Conversion/1 -> Relational Operator1/1
  Data Type Conversion1/1 -> Relational Operator2/1
  Unit Delay2/1 -> Switch/2
  Unit Delay/1 -> Data Type Conversion/1
  Governor/3(CrCtl_trqReqPWin_mp) -> CrCtl_trqReqPWin_mp/1
  Relational Operator1/1 -> EdgeRising/1, Governor/Enable
  EdgeRising/1 -> Governor/8(In1)
  In2/1 -> Governor/9(In2)

== system CrCtl_Governor/Acceleration State/CRCTL_SUBRMPEND ==
  GlbDa_aXFlt : Inport
  GlbDa_vXFlt : Inport  Port=2
  CrCtl_vMin : Inport  Port=3
  CrCtl_vMax : Inport  Port=4
  CrCtl_trqLimAct : Inport  Port=5
  CrCtl_trqMin : Inport  Port=6
  CrCtl_trqReqOld : Inport  Port=7
  Enable : EnablePort
  Add : Sum  Inputs=+-
  Constant : Constant  Value=ACC_ZERO
  Constant1 : Constant  Value=CrCtl_facAcc2TrqCor_C
  Logical Operator : Logic  Operator=OR  AllPortsSameDT=off  OutDataTypeStr=boolean
  Product : Product  OutDataTypeStr=Trq_Nm
  Relational Operator : RelationalOperator  Operator=<  OutDataTypeStr=boolean  RndMeth=Simplest
  Relational Operator1 : RelationalOperator  Operator=>  OutDataTypeStr=boolean  RndMeth=Simplest
  Relational Operator2 : RelationalOperator  Operator=<=  OutDataTypeStr=boolean  RndMeth=Simplest
  Saturation_S16 : CXLib/Saturation_S16
  Switch : Switch  Criteria=u2 ~= 0
  Switch1 : Switch  Criteria=u2 ~= 0
  Terminator : Terminator
  CrCtl_trqReq : Outport
  wires:
  GlbDa_vXFlt/1 -> Relational Operator1/1, Relational Operator/1
  CrCtl_vMin/1 -> Relational Operator/2
  CrCtl_vMax/1 -> Relational Operator1/2
  Relational Operator/1 -> Logical Operator/1
  Relational Operator1/1 -> Logical Operator/2
  GlbDa_aXFlt/1 -> Product/1, Relational Operator2/1
  Constant/1 -> Relational Operator2/2
  Constant1/1 -> Product/2
  Product/1 -> Add/2
  Add/1 -> Saturation_S16/1
  Relational Operator2/1 -> Switch/2
  Switch/1 -> Switch1/3
  Logical Operator/1 -> Switch1/2
  Saturation_S16/1 -> Switch/3
  Switch1/1 -> CrCtl_trqReq/1
  CrCtl_trqReqOld/1 -> Switch/1, Add/1, Switch1/1
  Saturation_S16/2 -> Terminator/1
  CrCtl_trqLimAct/1 -> Saturation_S16/3
  CrCtl_trqMin/1 -> Saturation_S16/2

== system CrCtl_Governor/Acceleration State/CRCTL_SUBSTRTVAL ==
  PT_rTraV2N : Inport
  WESDem_stCurr : Inport  Port=2
  VMD_trqDes : Inport  Port=3
  GlbDa_vXFlt : Inport  Port=4
  PT_trqWhl : Inport  Port=5
  CrCtl_trqLimAct : Inport  Port=6
  CrCtl_trqMin : Inport  Port=7
  Enable : EnablePort
  Add : Sum
  Add1 : Sum
  Constant : Constant  Value=WESDem_State_conv.WESDEM_STOFF
  Constant1 : Constant  Value=CrCtl_trqStrtAccOfs_C
  Constant2 : Constant  Value=CrCtl_facTrqStrtAcc_C
  MinMax : MinMax  Function=max  Inputs=2
  Product : Product  OutDataTypeStr=Trq_Nm
  Relational Operator : RelationalOperator  Operator=~=  OutDataTypeStr=boolean  RndMeth=Simplest
  Saturation_S16 : CXLib/Saturation_S16
  Switch : Switch  Criteria=u2 ~= 0
  Terminator : Terminator
  CrCtl_rTraV2NBeg : Outport
  CrCtl_trqReq : Outport  Port=2
  wires:
  PT_rTraV2N/1 -> CrCtl_rTraV2NBeg/1
  WESDem_stCurr/1 -> Relational Operator/1
  Constant/1 -> Relational Operator/2
  Relational Operator/1 -> Switch/2
  VMD_trqDes/1 -> Add/1
  Constant1/1 -> Add/2
  GlbDa_vXFlt/1 -> Product/1
  Constant2/1 -> Product/2
  Add/1 -> Add1/1
  Product/1 -> Add1/2
  Add1/1 -> MinMax/2, Switch/3
  PT_trqWhl/1 -> MinMax/1
  MinMax/1 -> Switch/1
  Switch/1 -> Saturation_S16/1
  CrCtl_trqMin/1 -> Saturation_S16/2
  CrCtl_trqLimAct/1 -> Saturation_S16/3
  Saturation_S16/2 -> Terminator/1
  Saturation_S16/1 -> CrCtl_trqReq/1

== system CrCtl_Governor/Acceleration State/CRCTL_SUBWAITRES ==
  PT_rTraV2N : Inport
  Enable : EnablePort
  CrCtl_rTraV2NBeg : Outport
  wires:
  PT_rTraV2N/1 -> CrCtl_rTraV2NBeg/1

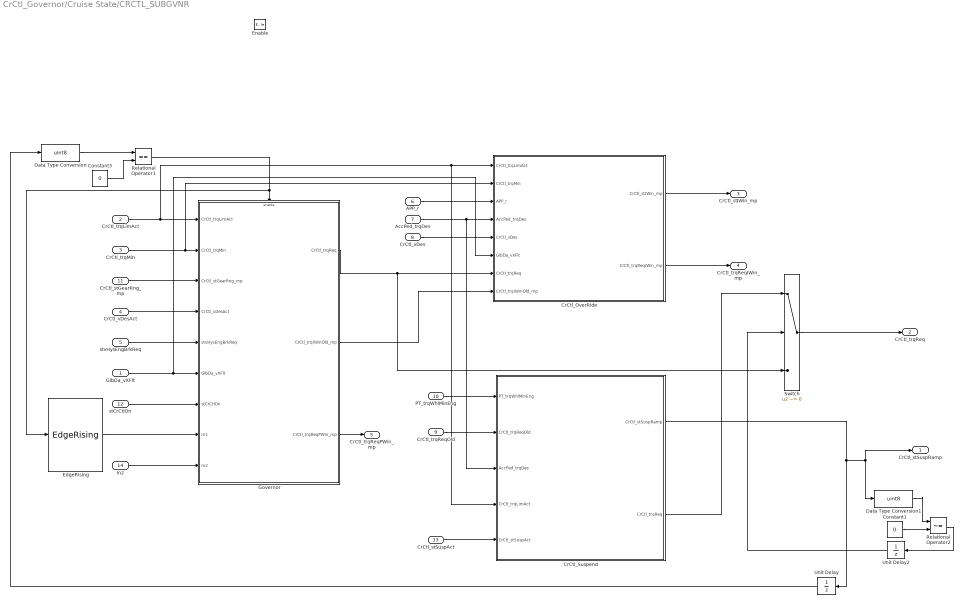
== system CrCtl_Governor/Cruise State/CRCTL_SUBGVNR ==
  GlbDa_vXFlt : Inport
  CrCtl_trqLimAct : Inport  Port=2
  CrCtl_trqMin : Inport  Port=3
  CrCtl_vDesAct : Inport  Port=4
  stvHysEngBrkReq : Inport  Port=5
  APP_r : Inport  Port=6
  AccPed_trqDes : Inport  Port=7
  CrCtl_vDes : Inport  Port=8
  CrCtl_trqReqOld : Inport  Port=9
  PT_trqWhlMinEng : Inport  Port=10
  CrCtl_stGearRng_mp : Inport  Port=11
  stCrCtlOn : Inport  Port=12
  CrCtl_stSuspAct : Inport  Port=13
  In2 : Inport  Port=14
  Enable : EnablePort
  Constant1 : Constant  Value=0  OutDataTypeStr=uint8
  Constant3 : Constant  Value=0  OutDataTypeStr=uint8
  CrCtl_OverRide : Subsystem
  CrCtl_Suspend : Subsystem
  Data Type Conversion : DataTypeConversion  OutDataTypeStr=uint8
  Data Type Conversion1 : DataTypeConversion  OutDataTypeStr=uint8
  EdgeRising : CXLib/EdgeRising
  Governor : Subsystem
  Relational Operator1 : RelationalOperator  Operator===  OutDataTypeStr=boolean  RndMeth=Simplest
  Relational Operator2 : RelationalOperator  Operator=~=  OutDataTypeStr=boolean  RndMeth=Simplest
  Switch : Switch  Criteria=u2 ~= 0
  Unit Delay : UnitDelay  InitialCondition=CrCtl_stSuspRamp_conv.CRCTL_SUSPENDNOTACTIVE  SampleTime=-1
  Unit Delay2 : UnitDelay  SampleTime=-1
  CrCtl_stSuspRamp : Outport
  CrCtl_trqReq : Outport  Port=2
  CrCtl_stIWin_mp : Outport  Port=3
  CrCtl_trqReqIWin_mp : Outport  Port=4
  CrCtl_trqReqPWin_mp : Outport  Port=5
  wires:
  Constant3/1 -> Relational Operator1/2
  stCrCtlOn/1 -> Governor/7(stCrCtlOn)
  stvHysEngBrkReq/1 -> Governor/5(stvHysEngBrkReq)
  CrCtl_vDesAct/1 -> Governor/4(CrCtl_vDesAct)
  CrCtl_stGearRng_mp/1 -> Governor/3(CrCtl_stGearRng_mp)
  CrCtl_trqMin/1 -> CrCtl_OverRide/2(CrCtl_trqMin), Governor/2(CrCtl_trqMin)
  APP_r/1 -> CrCtl_OverRide/3(APP_r)
  CrCtl_vDes/1 -> CrCtl_OverRide/5(CrCtl_vDes)
  GlbDa_vXFlt/1 -> Governor/6(GlbDa_vXFlt), CrCtl_OverRide/6(GlbDa_vXFlt)
  Governor/1(CrCtl_trqReq) -> Switch/3, CrCtl_OverRide/7(CrCtl_trqReq)
  Governor/2(CrCtl_trqIWinOld_mp) -> CrCtl_OverRide/8(CrCtl_trqIWinOld_mp)
  CrCtl_trqLimAct/1 -> Governor/1(CrCtl_trqLimAct), CrCtl_Suspend/4(CrCtl_trqLimAct), CrCtl_OverRide/1(CrCtl_trqLimAct)
  AccPed_trqDes/1 -> CrCtl_Suspend/3(AccPed_trqDes), CrCtl_OverRide/4(AccPed_trqDes)
  PT_trqWhlMinEng/1 -> CrCtl_Suspend/1(PT_trqWhlMinEng)
  CrCtl_trqReqOld/1 -> CrCtl_Suspend/2(CrCtl_trqReqOld)
  CrCtl_stSuspAct/1 -> CrCtl_Suspend/5(CrCtl_stSuspAct)
  CrCtl_Suspend/2(" CrCtl_trqReq") -> Switch/1
  CrCtl_Suspend/1(CrCtl_stSuspRamp) -> Unit Delay/1, CrCtl_stSuspRamp/1, Data Type Conversion1/1
  Switch/1 -> CrCtl_trqReq/1
  Constant1/1 -> Relational Operator2/2
  Relational Operator2/1 -> Unit Delay2/1
  CrCtl_OverRide/1(CrCtl_stIWin_mp) -> CrCtl_stIWin_mp/1
  CrCtl_OverRide/2(CrCtl_trqReqIWin_mp) -> CrCtl_trqReqIWin_mp/1
  Data Type Conversion/1 -> Relational Operator1/1
  Data Type Conversion1/1 -> Relational Operator2/1
  Unit Delay/1 -> Data Type Conversion/1
  Unit Delay2/1 -> Switch/2
  Governor/3(CrCtl_trqReqPWin_mp) -> CrCtl_trqReqPWin_mp/1
  Relational Operator1/1 -> EdgeRising/1, Governor/Enable
  EdgeRising/1 -> Governor/8(In1)
  In2/1 -> Governor/9(In2)

== system CrCtl_Governor/Cruise State/CRCTL_SUBSTRTVAL ==
  CrCtl_stGearRng_mp : Inport
  CrCtl_trqLimAct : Inport  Port=2
  CrCtl_trqMin : Inport  Port=3
  CrCtl_vDesAct : Inport  Port=4
  GlbDa_vXFlt : Inport  Port=5
  VMD_trqDes : Inport  Port=6
  Enable : EnablePort
  Add1 : Sum  Inputs=+-
  Add3 : Sum  Inputs=+-  OutDataTypeStr=Trq_Nm
  P_S16 : CXLib/P_S16
  Parameter Selection for Kp : Subsystem
  Saturation_S16 : CXLib/Saturation_S16
  Terminator : Terminator
  CrCtl_trqReq : Outport
  wires:
  CrCtl_vDesAct/1 -> Add1/1
  GlbDa_vXFlt/1 -> Add1/2
  CrCtl_stGearRng_mp/1 -> Parameter Selection for Kp/1(CrCtl_stGearRng_mp)
  Add1/1 -> P_S16/1
  P_S16/1 -> Add3/2
  Parameter Selection for Kp/1(Out1) -> P_S16/2
  Parameter Selection for Kp/2(Out2) -> P_S16/3
  Parameter Selection for Kp/3(Out3) -> P_S16/4
  Parameter Selection for Kp/4(Out4) -> P_S16/5
  Parameter Selection for Kp/5(Out5) -> P_S16/6
  Add3/1 -> Saturation_S16/1
  CrCtl_trqMin/1 -> Saturation_S16/2
  CrCtl_trqLimAct/1 -> Saturation_S16/3
  Saturation_S16/2 -> Terminator/1
  Saturation_S16/1 -> CrCtl_trqReq/1
  VMD_trqDes/1 -> Add3/1

== system CrCtl_Governor/Deceleration State/CRCTL_SUBPRECRUISE ==
  CrCtl_trqLimAct : Inport
  GlbDa_vXFlt : Inport  Port=2
  CrCtl_vDes : Inport  Port=3
  CrCtl_trqMin : Inport  Port=4
  CrCtl_vMaxDvtDecl : Inport  Port=5
  CrCtl_trqReq_Old : Inport  Port=6
  In1 : Inport  Port=7
  Enable : EnablePort
  Add : Sum  Inputs=+-
  Constant : Constant  Value=2  OutDataTypeStr=State_uint8
  Constant1 : Constant  Value=CrCtl_facRmpSlpHiDecl_C
  Constant2 : Constant  Value=CrCtl_swtTrqLimPreCruise_C
  Constant4 : Constant  Value=CrCtl_Governor_DT
  Logical Operator : Logic  Operator=OR  AllPortsSameDT=off  OutDataTypeStr=boolean
  Logical Operator1 : Logic  Operator=OR  AllPortsSameDT=off  OutDataTypeStr=boolean
  MinMax : MinMax  Function=max  Inputs=2
  Product : Product
  RAMP_S16 : CXLib/RAMP_S16
  Relational Operator : RelationalOperator  Operator=<=  OutDataTypeStr=boolean  RndMeth=Simplest
  Relational Operator1 : RelationalOperator  Operator=<=  OutDataTypeStr=boolean  RndMeth=Simplest
  Relational Operator2 : RelationalOperator  Operator===  OutDataTypeStr=boolean  RndMeth=Simplest
  Switch : Switch  Criteria=u2 ~= 0
  Switch1 : Switch  Criteria=u2 ~= 0
  Switch2 : Switch  Criteria=u2 ~= 0
  Unit Delay : UnitDelay  SampleTime=-1
  s2dt : CXLib/s2dt
  CrCtl_trqReq : Outport
  wires:
  Switch/1 -> s2dt/1
  Constant4/1 -> s2dt/2
  CrCtl_trqLimAct/1 -> Relational Operator2/2, RAMP_S16/1
  CrCtl_trqReq_Old/1 -> RAMP_S16/5
  CrCtl_vDes/1 -> Add/1
  CrCtl_vMaxDvtDecl/1 -> Add/2
  Add/1 -> Relational Operator/2
  GlbDa_vXFlt/1 -> Relational Operator/1
  Constant/1 -> Product/2
  Relational Operator/1 -> Switch/2
  Product/1 -> Switch/1
  Constant1/1 -> Switch/3, Product/1
  CrCtl_trqMin/1 -> Relational Operator1/2, MinMax/1
  MinMax/1 -> Switch1/3
  RAMP_S16/1 -> Relational Operator1/1, Relational Operator2/1, Switch1/1, MinMax/2
  Relational Operator1/1 -> Logical Operator/1
  Constant2/1 -> Switch2/2, Switch1/2
  Relational Operator2/1 -> Switch2/1, Logical Operator/2
  Logical Operator/1 -> Switch2/3
  Switch2/1 -> Unit Delay/1
  Logical Operator1/1 -> RAMP_S16/4
  Switch1/1 -> CrCtl_trqReq/1
  In1/1 -> Logical Operator1/1
  Unit Delay/1 -> Logical Operator1/2
  s2dt/1 -> RAMP_S16/3, RAMP_S16/2

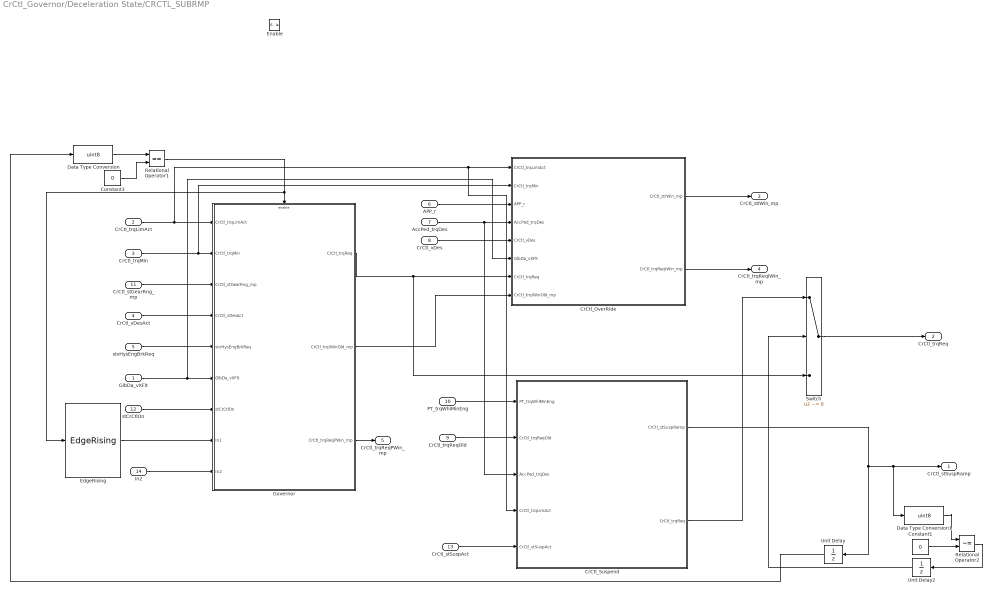
== system CrCtl_Governor/Deceleration State/CRCTL_SUBRMP ==
  GlbDa_vXFlt : Inport
  CrCtl_trqLimAct : Inport  Port=2
  CrCtl_trqMin : Inport  Port=3
  CrCtl_vDesAct : Inport  Port=4
  stvHysEngBrkReq : Inport  Port=5
  APP_r : Inport  Port=6
  AccPed_trqDes : Inport  Port=7
  CrCtl_vDes : Inport  Port=8
  CrCtl_trqReqOld : Inport  Port=9
  PT_trqWhlMinEng : Inport  Port=10
  CrCtl_stGearRng_mp : Inport  Port=11
  stCrCtlOn : Inport  Port=12
  CrCtl_stSuspAct : Inport  Port=13
  In2 : Inport  Port=14
  Enable : EnablePort
  Constant1 : Constant  Value=0  OutDataTypeStr=uint8
  Constant3 : Constant  Value=0  OutDataTypeStr=uint8
  CrCtl_OverRide : Subsystem
  CrCtl_Suspend : Subsystem
  Data Type Conversion : DataTypeConversion  OutDataTypeStr=uint8
  Data Type Conversion1 : DataTypeConversion  OutDataTypeStr=uint8
  EdgeRising : CXLib/EdgeRising
  Governor : Subsystem
  Relational Operator1 : RelationalOperator  Operator===  OutDataTypeStr=boolean  RndMeth=Simplest
  Relational Operator2 : RelationalOperator  Operator=~=  OutDataTypeStr=boolean  RndMeth=Simplest
  Switch : Switch  Criteria=u2 ~= 0
  Unit Delay : UnitDelay  InitialCondition=CrCtl_stSuspRamp_conv.CRCTL_SUSPENDNOTACTIVE  SampleTime=-1
  Unit Delay2 : UnitDelay  SampleTime=-1
  CrCtl_stSuspRamp : Outport
  CrCtl_trqReq : Outport  Port=2
  CrCtl_stIWin_mp : Outport  Port=3
  CrCtl_trqReqIWin_mp : Outport  Port=4
  CrCtl_trqReqPWin_mp : Outport  Port=5
  wires:
  Constant3/1 -> Relational Operator1/2
  stCrCtlOn/1 -> Governor/7(stCrCtlOn)
  stvHysEngBrkReq/1 -> Governor/5(stvHysEngBrkReq)
  CrCtl_vDesAct/1 -> Governor/4(CrCtl_vDesAct)
  CrCtl_stGearRng_mp/1 -> Governor/3(CrCtl_stGearRng_mp)
  CrCtl_trqMin/1 -> Governor/2(CrCtl_trqMin), CrCtl_OverRide/2(CrCtl_trqMin)
  APP_r/1 -> CrCtl_OverRide/3(APP_r)
  CrCtl_vDes/1 -> CrCtl_OverRide/5(CrCtl_vDes)
  GlbDa_vXFlt/1 -> Governor/6(GlbDa_vXFlt), CrCtl_OverRide/6(GlbDa_vXFlt)
  Governor/1(CrCtl_trqReq) -> Switch/3, CrCtl_OverRide/7(CrCtl_trqReq)
  Governor/2(CrCtl_trqIWinOld_mp) -> CrCtl_OverRide/8(CrCtl_trqIWinOld_mp)
  CrCtl_trqLimAct/1 -> Governor/1(CrCtl_trqLimAct), CrCtl_Suspend/4(CrCtl_trqLimAct), CrCtl_OverRide/1(CrCtl_trqLimAct)
  AccPed_trqDes/1 -> CrCtl_Suspend/3(AccPed_trqDes), CrCtl_OverRide/4(AccPed_trqDes)
  PT_trqWhlMinEng/1 -> CrCtl_Suspend/1(PT_trqWhlMinEng)
  CrCtl_trqReqOld/1 -> CrCtl_Suspend/2(CrCtl_trqReqOld)
  CrCtl_stSuspAct/1 -> CrCtl_Suspend/5(CrCtl_stSuspAct)
  CrCtl_Suspend/2(" CrCtl_trqReq") -> Switch/1
  CrCtl_Suspend/1(CrCtl_stSuspRamp) -> Unit Delay/1, Data Type Conversion1/1, CrCtl_stSuspRamp/1
  Switch/1 -> CrCtl_trqReq/1
  Constant1/1 -> Relational Operator2/2
  Relational Operator2/1 -> Unit Delay2/1
  CrCtl_OverRide/1(CrCtl_stIWin_mp) -> CrCtl_stIWin_mp/1
  CrCtl_OverRide/2(CrCtl_trqReqIWin_mp) -> CrCtl_trqReqIWin_mp/1
  Data Type Conversion/1 -> Relational Operator1/1
  Data Type Conversion1/1 -> Relational Operator2/1
  Unit Delay/1 -> Data Type Conversion/1
  Unit Delay2/1 -> Switch/2
  Governor/3(CrCtl_trqReqPWin_mp) -> CrCtl_trqReqPWin_mp/1
  Relational Operator1/1 -> EdgeRising/1, Governor/Enable
  EdgeRising/1 -> Governor/8(In1)
  In2/1 -> Governor/9(In2)

== system CrCtl_Governor/Deceleration State/CRCTL_SUBRMPEND ==
  GlbDa_aXFlt : Inport
  GlbDa_vXFlt : Inport  Port=2
  CrCtl_vMax : Inport  Port=3
  CrCtl_trqLimAct : Inport  Port=4
  CrCtl_trqMin : Inport  Port=5
  Enable : EnablePort
  Add : Sum
  Constant : Constant  Value=ACC_ZERO
  Constant1 : Constant  Value=CrCtl_facDecl2TrqCor_C
  Constant2 : Constant  Value=-1  OutDataTypeStr=int8
  MinMax : MinMax  Inputs=2  OutDataTypeStr=Acc_m_s2
  Product : Product  OutDataTypeStr=Trq_Nm
  Product1 : Product  OutDataTypeStr=Acc_m_s2
  Relational Operator1 : RelationalOperator  Operator=>  OutDataTypeStr=boolean  RndMeth=Simplest
  Saturation_S16 : CXLib/Saturation_S16
  Switch1 : Switch  Criteria=u2 ~= 0
  Terminator : Terminator
  Unit Delay : UnitDelay  SampleTime=-1
  CrCtl_trqReq : Outport
  wires:
  GlbDa_vXFlt/1 -> Relational Operator1/1
  CrCtl_vMax/1 -> Relational Operator1/2
  GlbDa_aXFlt/1 -> MinMax/1
  Constant1/1 -> Product/2
  Product/1 -> Add/2
  Add/1 -> Saturation_S16/1
  Saturation_S16/1 -> Switch1/3
  Relational Operator1/1 -> Switch1/2
  Switch1/1 -> Unit Delay/1, CrCtl_trqReq/1
  Saturation_S16/2 -> Terminator/1
  CrCtl_trqLimAct/1 -> Saturation_S16/3
  CrCtl_trqMin/1 -> Saturation_S16/2
  Constant/1 -> MinMax/2
  MinMax/1 -> Product1/1
  Unit Delay/1 -> Switch1/1, Add/1
  Product1/1 -> Product/1
  Constant2/1 -> Product1/2
